simulink model "Pi_si_perturbatii"  (R2022b)
settings: Solver=FixedStepAuto  StartTime=0.0  StopTime=2000  FixedStep=0.01  RelTol=1e-3
values from neighbouring files (symbols this model uses):
  C = 5.6    [CalculeProiect.m]
  h0 = 13.97    [CalculeProiect.m]
  h1 = 17.85    [CalculeProiect.m]
  k = 0.024    [CalculeProiect.m]
  k1 = 0.624    [CalculeProiect.m]
  k11 = k2*k2+4*(k-k3)*k1    (= 0.0616266)    [CalculeProiect.m]
  k12 = 8*(k-k3)    (= 0.1968)    [CalculeProiect.m]
  k13 = 2*(k-k3)    (= 0.0492)    [CalculeProiect.m]
  k2 = -0.015    [CalculeProiect.m]
  k3 = -0.0006    [CalculeProiect.m]
  kp = (delta_h/3)/delta_ua    (= 2.58666666667)    [CalculeProiect.m]
  q0 = 20.97    [CalculeProiect.m]
undefined symbols (not defined in the file or in its folder): ki
libraries: slpidlib x3
settings Model: Creator=denis  LastModifiedBy=denis

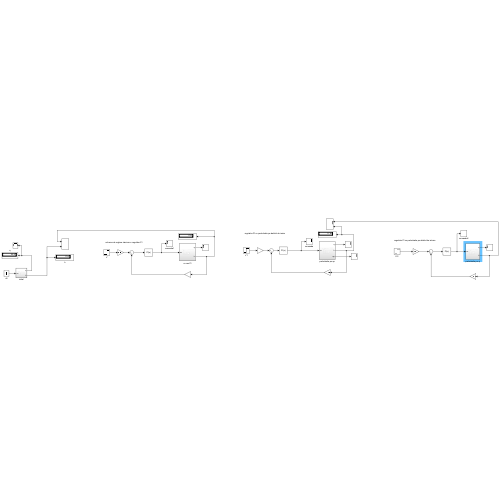
[thumbnail: Simulink's stored preview of the top-level diagram]
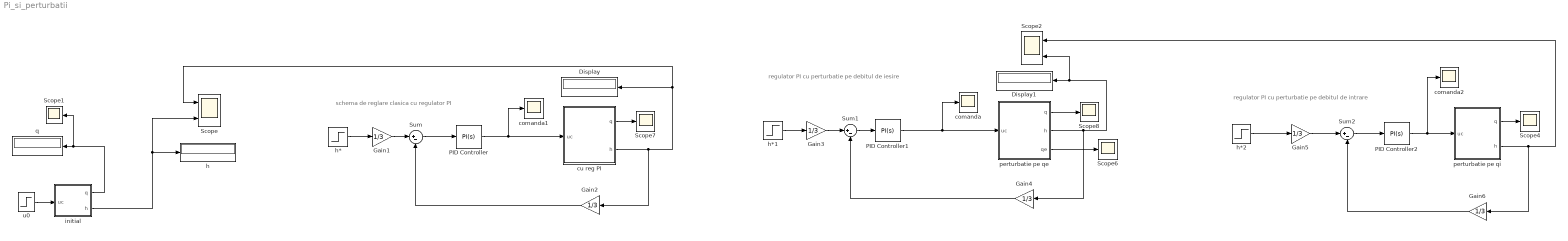
== system Pi_si_perturbatii ==
  note: schema de reglare clasica cu regulator PI
  note: regulator PI cu perturbatie pe debitul de iesire
  note: regulator PI cu perturbatie pe debitul de intrare
  Display : Display
  Display1 : Display
  Gain{1..6} (6 alike) : Gain  Gain=1/3
  PID Controller : slpidlib/PID Controller  Controller=PI  Form=Parallel  TimeDomain=Continuous-time  UseExternalTs=off  SampleTime=-1  IntegratorMethod=Forward Euler  FilterMethod=Forward Euler  ControllerParametersSource=internal  P=kp  I=ki  UseKiTs=off  D=0  N=100  UseFilter=on  TunerSelectOption=Transfer Function Based (PID Tuner App)  InitialConditionSource=internal  InitialConditionForIntegrator=4.4  InitialConditionForFilter=0  DifferentiatorICPrevScaledInput=0  ExternalReset=none  TrackingMode=off  Kt=1  LimitOutput=off  SatLimitsSource=internal  UpperSaturationLimit=inf  LowerSaturationLimit=-inf  LinearizeAsGain=on  AntiWindupMode=none  Kb=1  LimitIntegrator=off  UpperIntegratorSaturationLimit=inf  LowerIntegratorSaturationLimit=-inf  POutMin=[]  POutMax=[]  IOutMin=[]  IOutMax=[]  DOutMin=[]  DOutMax=[]  NOutMin=[]  NOutMax=[]  SumOutMin=[]  SumOutMax=[]  SaturationOutMin=[]  SaturationOutMax=[]  PParamMin=[]  PParamMax=[]  IParamMin=[]  IParamMax=[]  DParamMin=[]  DParamMax=[]  NParamMin=[]  NParamMax=[]  KbParamMin=[]  KbParamMax=[]  KtParamMin=[]  KtParamMax=[]  KbOutMin=[]  KbOutMax=[]  KtOutMin=[]  KtOutMax=[]  IntegratorOutMin=[]  IntegratorOutMax=[]  FilterOutMin=[]  FilterOutMax=[]  SumI1OutMin=[]  SumI1OutMax=[]  SumI2OutMin=[]  SumI2OutMax=[]  SumI3OutMin=[]  SumI3OutMax=[]  SumI4OutMin=[]  SumI4OutMax=[]  SumDOutMin=[]  SumDOutMax=[]  DifferentiatorOutMin=[]  DifferentiatorOutMax=[]  FilterDiffOutCoefMin=[]  FilterDiffOutCoefMax=[]  ReciprocalOutMin=[]  ReciprocalOutMax=[]  SumDenOutMin=[]  SumDenOutMax=[]  SumNumOutMin=[]  SumNumOutMax=[]  DivideOutMin=[]  DivideOutMax=[]  UdiffTsProdOutMin=[]  UdiffTsProdOutMax=[]  NTsProdOutMin=[]  NTsProdOutMax=[]  UintegralTsProdOutMin=[]  UintegralTsProdOutMax=[]  UngainTsProdOutMin=[]  UngainTsProdOutMax=[]  ClampingZeroOutDataTypeStr=Inherit: Inherit via back propagation  ClampingZeroOutMin=[]  ClampingZeroOutMax=[]  FilterDenConstantOutDataTypeStr=Inherit: Inherit via back propagation  FilterDenConstantOutMin=[]  FilterDenConstantOutMax=[]  PCopyOutDataTypeStr=Inherit: Inherit via back propagation  PCopyOutMin=[]  PCopyOutMax=[]  NCopyOutDataTypeStr=Inherit: Inherit via back propagation  NCopyOutMin=[]  NCopyOutMax=[]  IntegratorContinuousStateAttributes=''  IntegratorStateMustResolveToSignalObject=off  IntegratorRTWStateStorageClass=Auto  FilterContinuousStateAttributes=''  FilterStateMustResolveToSignalObject=off  FilterRTWStateStorageClass=Auto  ParallelPVariant=InternalParameters  IdealPVariant=Disabled  IVariant=InternalParameters  DVariant=Disabled  IntegratorVariant=Continuous  SatVariant=Disabled  AWVariant=Passthrough  PCopyVariant=Disabled  TRVariant=Disabled  FdbkBlocksVariant=Forward  IdealPFdbkVariant=Disabled  SatFdbkVariant=Disabled  DerivativeFilterVariant=Disabled  NVariant=Disabled  NCopyVariant=Disabled_SignalSpec  FilterICVariant=Disabled  IntegratorICVariant=InternalICs  ExternalResetVariant=Disabled  TRSumVariant=Passthrough  SumFdbkVariant=Disabled  SumVariant=Sum_PI  TsampFilterVariant=InternalTs  TsampNgainVariant=Passthrough  TsampIntegralVariant=Passthrough  ExternalSaturationOutDataTypeStr=Inherit: Same as second input
  PID Controller1 : slpidlib/PID Controller  Controller=PI  Form=Parallel  TimeDomain=Continuous-time  UseExternalTs=off  SampleTime=-1  IntegratorMethod=Forward Euler  FilterMethod=Forward Euler  ControllerParametersSource=internal  P=kp  I=ki  UseKiTs=off  D=0  N=100  UseFilter=on  TunerSelectOption=Transfer Function Based (PID Tuner App)  InitialConditionSource=internal  InitialConditionForIntegrator=4.4  InitialConditionForFilter=0  DifferentiatorICPrevScaledInput=0  ExternalReset=none  TrackingMode=off  Kt=1  LimitOutput=off  SatLimitsSource=internal  UpperSaturationLimit=inf  LowerSaturationLimit=-inf  LinearizeAsGain=on  AntiWindupMode=none  Kb=1  LimitIntegrator=off  UpperIntegratorSaturationLimit=inf  LowerIntegratorSaturationLimit=-inf  POutMin=[]  POutMax=[]  IOutMin=[]  IOutMax=[]  DOutMin=[]  DOutMax=[]  NOutMin=[]  NOutMax=[]  SumOutMin=[]  SumOutMax=[]  SaturationOutMin=[]  SaturationOutMax=[]  PParamMin=[]  PParamMax=[]  IParamMin=[]  IParamMax=[]  DParamMin=[]  DParamMax=[]  NParamMin=[]  NParamMax=[]  KbParamMin=[]  KbParamMax=[]  KtParamMin=[]  KtParamMax=[]  KbOutMin=[]  KbOutMax=[]  KtOutMin=[]  KtOutMax=[]  IntegratorOutMin=[]  IntegratorOutMax=[]  FilterOutMin=[]  FilterOutMax=[]  SumI1OutMin=[]  SumI1OutMax=[]  SumI2OutMin=[]  SumI2OutMax=[]  SumI3OutMin=[]  SumI3OutMax=[]  SumI4OutMin=[]  SumI4OutMax=[]  SumDOutMin=[]  SumDOutMax=[]  DifferentiatorOutMin=[]  DifferentiatorOutMax=[]  FilterDiffOutCoefMin=[]  FilterDiffOutCoefMax=[]  ReciprocalOutMin=[]  ReciprocalOutMax=[]  SumDenOutMin=[]  SumDenOutMax=[]  SumNumOutMin=[]  SumNumOutMax=[]  DivideOutMin=[]  DivideOutMax=[]  UdiffTsProdOutMin=[]  UdiffTsProdOutMax=[]  NTsProdOutMin=[]  NTsProdOutMax=[]  UintegralTsProdOutMin=[]  UintegralTsProdOutMax=[]  UngainTsProdOutMin=[]  UngainTsProdOutMax=[]  ClampingZeroOutDataTypeStr=Inherit: Inherit via back propagation  ClampingZeroOutMin=[]  ClampingZeroOutMax=[]  FilterDenConstantOutDataTypeStr=Inherit: Inherit via back propagation  FilterDenConstantOutMin=[]  FilterDenConstantOutMax=[]  PCopyOutDataTypeStr=Inherit: Inherit via back propagation  PCopyOutMin=[]  PCopyOutMax=[]  NCopyOutDataTypeStr=Inherit: Inherit via back propagation  NCopyOutMin=[]  NCopyOutMax=[]  IntegratorContinuousStateAttributes=''  IntegratorStateMustResolveToSignalObject=off  IntegratorRTWStateStorageClass=Auto  FilterContinuousStateAttributes=''  FilterStateMustResolveToSignalObject=off  FilterRTWStateStorageClass=Auto  ParallelPVariant=InternalParameters  IdealPVariant=Disabled  IVariant=InternalParameters  DVariant=Disabled  IntegratorVariant=Continuous  SatVariant=Disabled  AWVariant=Passthrough  PCopyVariant=Disabled  TRVariant=Disabled  FdbkBlocksVariant=Forward  IdealPFdbkVariant=Disabled  SatFdbkVariant=Disabled  DerivativeFilterVariant=Disabled  NVariant=Disabled  NCopyVariant=Disabled_SignalSpec  FilterICVariant=Disabled  IntegratorICVariant=InternalICs  ExternalResetVariant=Disabled  TRSumVariant=Passthrough  SumFdbkVariant=Disabled  SumVariant=Sum_PI  TsampFilterVariant=InternalTs  TsampNgainVariant=Passthrough  TsampIntegralVariant=Passthrough  ExternalSaturationOutDataTypeStr=Inherit: Same as second input
  PID Controller2 : slpidlib/PID Controller  Controller=PI  Form=Parallel  TimeDomain=Continuous-time  UseExternalTs=off  SampleTime=-1  IntegratorMethod=Forward Euler  FilterMethod=Forward Euler  ControllerParametersSource=internal  P=kp  I=ki  UseKiTs=off  D=0  N=100  UseFilter=on  TunerSelectOption=Transfer Function Based (PID Tuner App)  InitialConditionSource=internal  InitialConditionForIntegrator=4.4  InitialConditionForFilter=0  DifferentiatorICPrevScaledInput=0  ExternalReset=none  TrackingMode=off  Kt=1  LimitOutput=off  SatLimitsSource=internal  UpperSaturationLimit=inf  LowerSaturationLimit=-inf  LinearizeAsGain=on  AntiWindupMode=none  Kb=1  LimitIntegrator=off  UpperIntegratorSaturationLimit=inf  LowerIntegratorSaturationLimit=-inf  POutMin=[]  POutMax=[]  IOutMin=[]  IOutMax=[]  DOutMin=[]  DOutMax=[]  NOutMin=[]  NOutMax=[]  SumOutMin=[]  SumOutMax=[]  SaturationOutMin=[]  SaturationOutMax=[]  PParamMin=[]  PParamMax=[]  IParamMin=[]  IParamMax=[]  DParamMin=[]  DParamMax=[]  NParamMin=[]  NParamMax=[]  KbParamMin=[]  KbParamMax=[]  KtParamMin=[]  KtParamMax=[]  KbOutMin=[]  KbOutMax=[]  KtOutMin=[]  KtOutMax=[]  IntegratorOutMin=[]  IntegratorOutMax=[]  FilterOutMin=[]  FilterOutMax=[]  SumI1OutMin=[]  SumI1OutMax=[]  SumI2OutMin=[]  SumI2OutMax=[]  SumI3OutMin=[]  SumI3OutMax=[]  SumI4OutMin=[]  SumI4OutMax=[]  SumDOutMin=[]  SumDOutMax=[]  DifferentiatorOutMin=[]  DifferentiatorOutMax=[]  FilterDiffOutCoefMin=[]  FilterDiffOutCoefMax=[]  ReciprocalOutMin=[]  ReciprocalOutMax=[]  SumDenOutMin=[]  SumDenOutMax=[]  SumNumOutMin=[]  SumNumOutMax=[]  DivideOutMin=[]  DivideOutMax=[]  UdiffTsProdOutMin=[]  UdiffTsProdOutMax=[]  NTsProdOutMin=[]  NTsProdOutMax=[]  UintegralTsProdOutMin=[]  UintegralTsProdOutMax=[]  UngainTsProdOutMin=[]  UngainTsProdOutMax=[]  ClampingZeroOutDataTypeStr=Inherit: Inherit via back propagation  ClampingZeroOutMin=[]  ClampingZeroOutMax=[]  FilterDenConstantOutDataTypeStr=Inherit: Inherit via back propagation  FilterDenConstantOutMin=[]  FilterDenConstantOutMax=[]  PCopyOutDataTypeStr=Inherit: Inherit via back propagation  PCopyOutMin=[]  PCopyOutMax=[]  NCopyOutDataTypeStr=Inherit: Inherit via back propagation  NCopyOutMin=[]  NCopyOutMax=[]  IntegratorContinuousStateAttributes=''  IntegratorStateMustResolveToSignalObject=off  IntegratorRTWStateStorageClass=Auto  FilterContinuousStateAttributes=''  FilterStateMustResolveToSignalObject=off  FilterRTWStateStorageClass=Auto  ParallelPVariant=InternalParameters  IdealPVariant=Disabled  IVariant=InternalParameters  DVariant=Disabled  IntegratorVariant=Continuous  SatVariant=Disabled  AWVariant=Passthrough  PCopyVariant=Disabled  TRVariant=Disabled  FdbkBlocksVariant=Forward  IdealPFdbkVariant=Disabled  SatFdbkVariant=Disabled  DerivativeFilterVariant=Disabled  NVariant=Disabled  NCopyVariant=Disabled_SignalSpec  FilterICVariant=Disabled  IntegratorICVariant=InternalICs  ExternalResetVariant=Disabled  TRSumVariant=Passthrough  SumFdbkVariant=Disabled  SumVariant=Sum_PI  TsampFilterVariant=InternalTs  TsampNgainVariant=Passthrough  TsampIntegralVariant=Passthrough  ExternalSaturationOutDataTypeStr=Inherit: Same as second input
  Scope : Scope  NumInputPorts=2
  Scope{1,4,6..8} (5 alike) : Scope
  Scope2 : Scope  NumInputPorts=2
  Sum : Sum  Inputs=|+-
  Sum1 : Sum  Inputs=|+-
  Sum2 : Sum  Inputs=|+-
  comanda : Scope
  comanda1 : Scope
  comanda2 : Scope
  cu reg PI : Subsystem
  h : Display
  h* : Step  Time=0  Before=h0  After=h1  SampleTime=0
  h*1 : Step  Time=0  Before=h0  After=h1  SampleTime=0
  h*2 : Step  Time=0  Before=h0  After=h1  SampleTime=0
  initial : Subsystem
  perturbatie pe qe : Subsystem
  perturbatie pe qi : Subsystem
  q : Display
  u0 : Step  Time=0  Before=4.4  After=4.9  SampleTime=0
  wires:
  Sum2/1 -> PID Controller2/1
  h*2/1 -> Gain5/1
  perturbatie pe qe/1(q) -> Scope8/1
  perturbatie pe qi/1(q) -> Scope4/1
  Gain5/1 -> Sum2/1
  Gain3/1 -> Sum1/1
  initial/2(h) -> Scope/2, h/1
  Sum/1 -> PID Controller/1
  Sum1/1 -> PID Controller1/1
  PID Controller/1 -> comanda1/1, cu reg PI/1(uc)
  h*1/1 -> Gain3/1
  Gain6/1 -> Sum2/2
  perturbatie pe qe/2(h) -> Gain4/1, Scope2/2, Display1/1
  PID Controller1/1 -> comanda/1, perturbatie pe qe/1(uc)
  Gain4/1 -> Sum1/2
  perturbatie pe qe/3(qe) -> Scope6/1
  h*/1 -> Gain1/1
  Gain2/1 -> Sum/2
  perturbatie pe qi/2(h) -> Scope2/1, Gain6/1
  u0/1 -> initial/1(uc)
  cu reg PI/2(h) -> Gain2/1, Display/1, Scope/1
  cu reg PI/1(q) -> Scope7/1
  Gain1/1 -> Sum/1
  PID Controller2/1 -> comanda2/1, perturbatie pe qi/1(uc)
  initial/1(q) -> Scope1/1, q/1

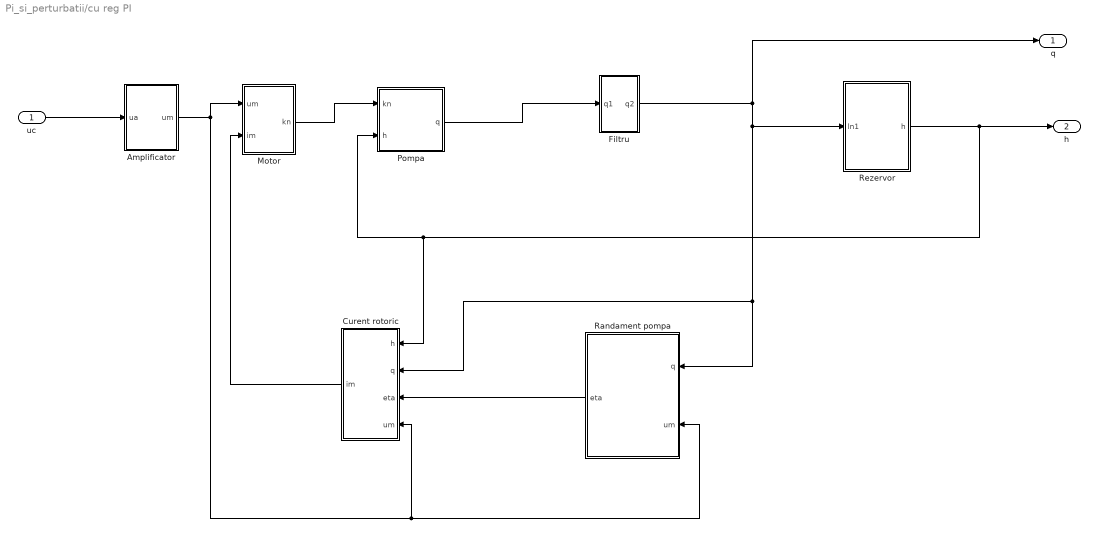
== system Pi_si_perturbatii/cu reg PI ==
  uc : Inport
  Amplificator : Subsystem
  Curent rotoric : Subsystem
  Filtru : Subsystem
  Motor : Subsystem
  Pompa : Subsystem
  Randament pompa : Subsystem
  Rezervor : Subsystem
  q : Outport
  h : Outport  Port=2
  wires:
  Filtru/1(q2) -> Curent rotoric/2(q), Randament pompa/1(q), Rezervor/1(ln1), q/1
  Rezervor/1(h) -> h/1, Curent rotoric/1(h), Pompa/2(h)
  Motor/1(kn) -> Pompa/1(kn)
  Curent rotoric/1(im) -> Motor/2(im)
  Amplificator/1(um) -> Motor/1(um), Curent rotoric/4(um), Randament pompa/2(um)
  uc/1 -> Amplificator/1(ua)
  Randament pompa/1(eta) -> Curent rotoric/3(eta)
  Pompa/1(q) -> Filtru/1(q1)

== system Pi_si_perturbatii/initial ==
  uc : Inport
  Amplificator : Subsystem
  Curent rotoric : Subsystem
  Filtru : Subsystem
  Motor : Subsystem
  Pompa : Subsystem
  Randament pompa : Subsystem
  Rezervor : Subsystem
  q : Outport
  h : Outport  Port=2
  wires:
  Filtru/1(q2) -> Curent rotoric/2(q), Randament pompa/1(q), Rezervor/1(ln1), q/1
  Rezervor/1(h) -> h/1, Curent rotoric/1(h), Pompa/2(h)
  Motor/1(kn) -> Pompa/1(kn)
  Curent rotoric/1(im) -> Motor/2(im)
  Amplificator/1(um) -> Motor/1(um), Curent rotoric/4(um), Randament pompa/2(um)
  uc/1 -> Amplificator/1(ua)
  Randament pompa/1(eta) -> Curent rotoric/3(eta)
  Pompa/1(q) -> Filtru/1(q1)

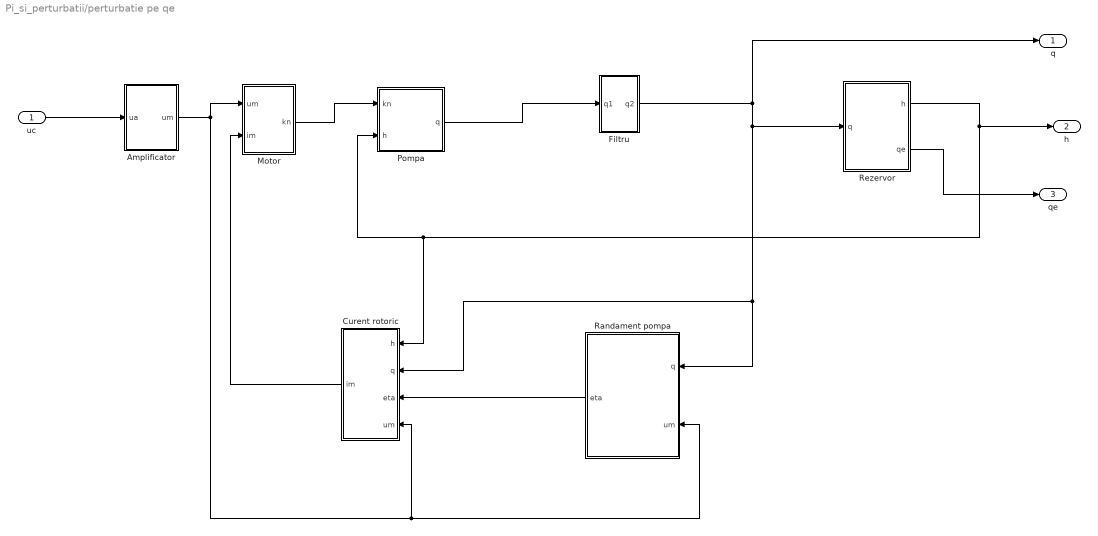
== system Pi_si_perturbatii/perturbatie pe qe ==
  uc : Inport
  Amplificator : Subsystem
  Curent rotoric : Subsystem
  Filtru : Subsystem
  Motor : Subsystem
  Pompa : Subsystem
  Randament pompa : Subsystem
  Rezervor : Subsystem
  q : Outport
  h : Outport  Port=2
  qe : Outport  Port=3
  wires:
  Filtru/1(q2) -> Curent rotoric/2(q), Randament pompa/1(q), Rezervor/1(q), q/1
  Rezervor/1(h) -> h/1, Curent rotoric/1(h), Pompa/2(h)
  Motor/1(kn) -> Pompa/1(kn)
  Curent rotoric/1(im) -> Motor/2(im)
  Amplificator/1(um) -> Motor/1(um), Curent rotoric/4(um), Randament pompa/2(um)
  uc/1 -> Amplificator/1(ua)
  Randament pompa/1(eta) -> Curent rotoric/3(eta)
  Pompa/1(q) -> Filtru/1(q1)
  Rezervor/2(qe) -> qe/1

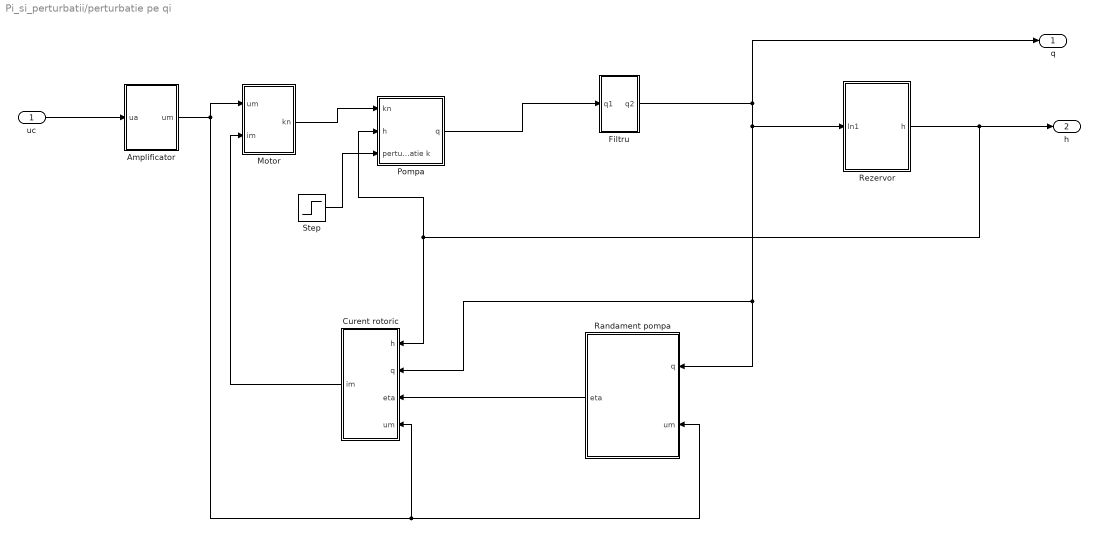
== system Pi_si_perturbatii/perturbatie pe qi ==
  uc : Inport
  Amplificator : Subsystem
  Curent rotoric : Subsystem
  Filtru : Subsystem
  Motor : Subsystem
  Pompa : Subsystem
  Randament pompa : Subsystem
  Rezervor : Subsystem
  Step : Step  Time=250  After=0.03  SampleTime=0
  q : Outport
  h : Outport  Port=2
  wires:
  Filtru/1(q2) -> Curent rotoric/2(q), Randament pompa/1(q), Rezervor/1(ln1), q/1
  Rezervor/1(h) -> h/1, Pompa/2(h), Curent rotoric/1(h)
  Motor/1(kn) -> Pompa/1(kn)
  Curent rotoric/1(im) -> Motor/2(im)
  Amplificator/1(um) -> Motor/1(um), Curent rotoric/4(um), Randament pompa/2(um)
  uc/1 -> Amplificator/1(ua)
  Randament pompa/1(eta) -> Curent rotoric/3(eta)
  Pompa/1(q) -> Filtru/1(q1)
  Step/1 -> Pompa/3(perturbatie k)

== system Pi_si_perturbatii/cu reg PI/Amplificator ==
  ua : Inport
  Constant : Constant  Value=8.1
  Gain : Gain  Gain=2.2
  Gain1 : Gain  Gain=5
  Gain2 : Gain  Gain=2.2
  Saturation : Saturate  UpperLimit=22  LowerLimit=0
  Sum : Sum  Inputs=|++
  Sum1 : Sum  Inputs=|+-
  Switch : Switch  Criteria=u2 > Threshold  Threshold=8.1  SaturateOnIntegerOverflow=off  InputSameDT=off
  um : Outport
  wires:
  Gain/1 -> Switch/3
  Sum1/1 -> Gain1/1
  ua/1 -> Gain/1, Sum1/1, Gain2/1, Switch/2
  Switch/1 -> Saturation/1
  Gain1/1 -> Sum/2
  Saturation/1 -> um/1
  Constant/1 -> Sum1/2
  Gain2/1 -> Sum/1
  Sum/1 -> Switch/1

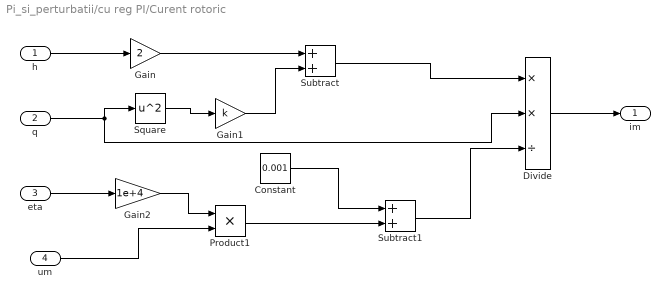
== system Pi_si_perturbatii/cu reg PI/Curent rotoric ==
  h : Inport
  q : Inport  Port=2
  eta : Inport  Port=3
  um : Inport  Port=4
  Constant : Constant  Value=0.001
  Divide : Product  Inputs=**/
  Gain : Gain  Gain=2
  Gain1 : Gain  Gain=k
  Gain2 : Gain  Gain=1e+4
  Product1 : Product
  Square : Math  Operator=square
  Subtract : Sum
  Subtract1 : Sum
  im : Outport
  wires:
  h/1 -> Gain/1
  Divide/1 -> im/1
  q/1 -> Divide/2, Square/1
  eta/1 -> Gain2/1
  um/1 -> Product1/2
  Gain2/1 -> Product1/1
  Subtract/1 -> Divide/1
  Constant/1 -> Subtract1/1
  Product1/1 -> Subtract1/2
  Subtract1/1 -> Divide/3
  Gain/1 -> Subtract/1
  Gain1/1 -> Subtract/2
  Square/1 -> Gain1/1

== system Pi_si_perturbatii/cu reg PI/Filtru ==
  q1 : Inport
  Integrator1 : Integrator  InitialCondition=q0
  Sum1 : Sum  Inputs=|+-
  q2 : Outport
  wires:
  Integrator1/1 -> q2/1, Sum1/2
  q1/1 -> Sum1/1
  Sum1/1 -> Integrator1/1

== system Pi_si_perturbatii/cu reg PI/Motor ==
  um : Inport
  im : Inport  Port=2
  Add : Sum  Inputs=+-
  Rm : Gain  Gain=3
  kn : Outport
  wires:
  Rm/1 -> Add/2
  um/1 -> Add/1
  im/1 -> Rm/1
  Add/1 -> kn/1

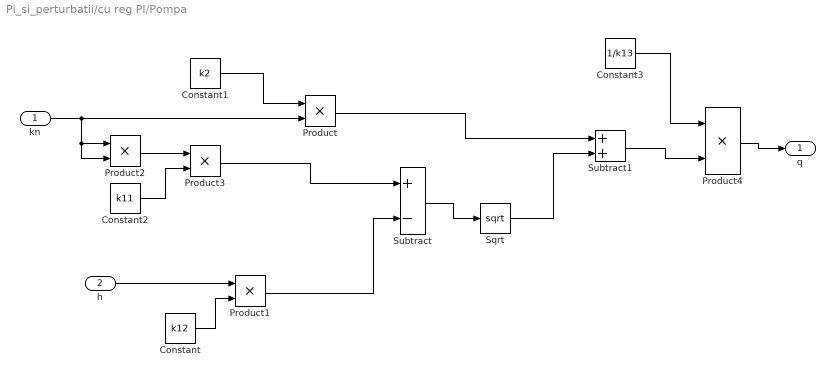
== system Pi_si_perturbatii/cu reg PI/Pompa ==
  kn : Inport
  h : Inport  Port=2
  Constant : Constant  Value=k12
  Constant1 : Constant  Value=k2
  Constant2 : Constant  Value=k11
  Constant3 : Constant  Value=1/k13
  Product{,1..4} (5 alike) : Product
  Sqrt : Sqrt
  Subtract : Sum  Inputs=+-
  Subtract1 : Sum
  q : Outport
  wires:
  Subtract/1 -> Sqrt/1
  Sqrt/1 -> Subtract1/2
  h/1 -> Product1/1
  Product1/1 -> Subtract/2
  Constant/1 -> Product1/2
  Constant1/1 -> Product/1
  kn/1 -> Product2/2, Product2/1, Product/2
  Product/1 -> Subtract1/1
  Product2/1 -> Product3/1
  Constant2/1 -> Product3/2
  Product3/1 -> Subtract/1
  Constant3/1 -> Product4/1
  Subtract1/1 -> Product4/2
  Product4/1 -> q/1

== system Pi_si_perturbatii/cu reg PI/Randament pompa ==
  q : Inport
  um : Inport  Port=2
  Gain : Gain  Gain=8e-5
  Product : Product
  eta : Outport
  wires:
  um/1 -> Gain/1
  Gain/1 -> Product/2
  q/1 -> Product/1
  Product/1 -> eta/1

== system Pi_si_perturbatii/cu reg PI/Rezervor ==
  ln1 : Inport
  Gain : Gain  Gain=1/332.5
  Gain1 : Gain  Gain=C
  Integrator1 : Integrator  InitialCondition=h0
  Sqrt : Sqrt
  Sum1 : Sum  Inputs=|+-
  h : Outport
  wires:
  Gain/1 -> Integrator1/1
  Integrator1/1 -> Sqrt/1, h/1
  Sum1/1 -> Gain/1
  ln1/1 -> Sum1/1
  Sqrt/1 -> Gain1/1
  Gain1/1 -> Sum1/2

== system Pi_si_perturbatii/initial/Amplificator ==
  ua : Inport
  Constant : Constant  Value=8.1
  Gain : Gain  Gain=2.2
  Gain1 : Gain  Gain=5
  Gain2 : Gain  Gain=2.2
  Saturation : Saturate  UpperLimit=22  LowerLimit=0
  Sum : Sum  Inputs=|++
  Sum1 : Sum  Inputs=|+-
  Switch : Switch  Criteria=u2 > Threshold  Threshold=8.1  SaturateOnIntegerOverflow=off  InputSameDT=off
  um : Outport
  wires:
  Gain/1 -> Switch/3
  Sum1/1 -> Gain1/1
  ua/1 -> Gain/1, Sum1/1, Gain2/1, Switch/2
  Switch/1 -> Saturation/1
  Gain1/1 -> Sum/2
  Saturation/1 -> um/1
  Constant/1 -> Sum1/2
  Gain2/1 -> Sum/1
  Sum/1 -> Switch/1

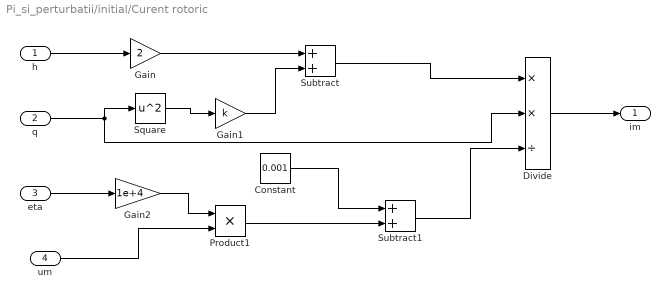
== system Pi_si_perturbatii/initial/Curent rotoric ==
  h : Inport
  q : Inport  Port=2
  eta : Inport  Port=3
  um : Inport  Port=4
  Constant : Constant  Value=0.001
  Divide : Product  Inputs=**/
  Gain : Gain  Gain=2
  Gain1 : Gain  Gain=k
  Gain2 : Gain  Gain=1e+4
  Product1 : Product
  Square : Math  Operator=square
  Subtract : Sum
  Subtract1 : Sum
  im : Outport
  wires:
  h/1 -> Gain/1
  Divide/1 -> im/1
  q/1 -> Divide/2, Square/1
  eta/1 -> Gain2/1
  um/1 -> Product1/2
  Gain2/1 -> Product1/1
  Subtract/1 -> Divide/1
  Constant/1 -> Subtract1/1
  Product1/1 -> Subtract1/2
  Subtract1/1 -> Divide/3
  Gain/1 -> Subtract/1
  Gain1/1 -> Subtract/2
  Square/1 -> Gain1/1

== system Pi_si_perturbatii/initial/Filtru ==
  q1 : Inport
  Integrator1 : Integrator  InitialCondition=q0
  Sum1 : Sum  Inputs=|+-
  q2 : Outport
  wires:
  Integrator1/1 -> q2/1, Sum1/2
  q1/1 -> Sum1/1
  Sum1/1 -> Integrator1/1

== system Pi_si_perturbatii/initial/Motor ==
  um : Inport
  im : Inport  Port=2
  Add : Sum  Inputs=+-
  Rm : Gain  Gain=3
  kn : Outport
  wires:
  Rm/1 -> Add/2
  um/1 -> Add/1
  im/1 -> Rm/1
  Add/1 -> kn/1

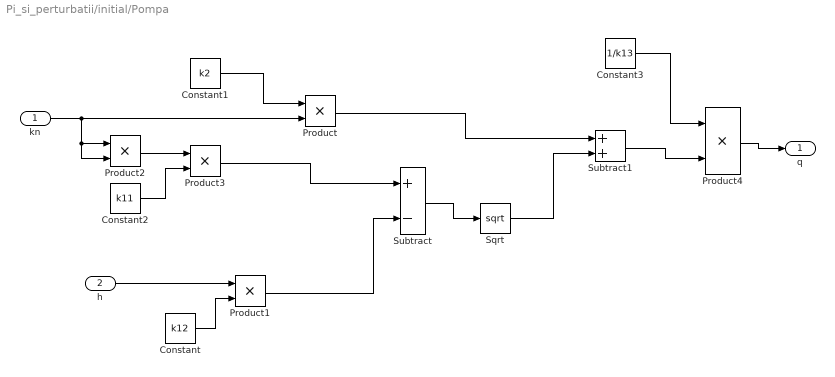
== system Pi_si_perturbatii/initial/Pompa ==
  kn : Inport
  h : Inport  Port=2
  Constant : Constant  Value=k12
  Constant1 : Constant  Value=k2
  Constant2 : Constant  Value=k11
  Constant3 : Constant  Value=1/k13
  Product{,1..4} (5 alike) : Product
  Sqrt : Sqrt
  Subtract : Sum  Inputs=+-
  Subtract1 : Sum
  q : Outport
  wires:
  Subtract/1 -> Sqrt/1
  Sqrt/1 -> Subtract1/2
  h/1 -> Product1/1
  Product1/1 -> Subtract/2
  Constant/1 -> Product1/2
  Constant1/1 -> Product/1
  kn/1 -> Product2/2, Product2/1, Product/2
  Product/1 -> Subtract1/1
  Product2/1 -> Product3/1
  Constant2/1 -> Product3/2
  Product3/1 -> Subtract/1
  Constant3/1 -> Product4/1
  Subtract1/1 -> Product4/2
  Product4/1 -> q/1

== system Pi_si_perturbatii/initial/Randament pompa ==
  q : Inport
  um : Inport  Port=2
  Gain : Gain  Gain=8e-5
  Product : Product
  eta : Outport
  wires:
  um/1 -> Gain/1
  Gain/1 -> Product/2
  q/1 -> Product/1
  Product/1 -> eta/1

== system Pi_si_perturbatii/initial/Rezervor ==
  ln1 : Inport
  Gain : Gain  Gain=1/332.5
  Gain1 : Gain  Gain=C
  Integrator1 : Integrator  InitialCondition=h0
  Sqrt : Sqrt
  Sum1 : Sum  Inputs=|+-
  h : Outport
  wires:
  Gain/1 -> Integrator1/1
  Integrator1/1 -> Sqrt/1, h/1
  Sum1/1 -> Gain/1
  ln1/1 -> Sum1/1
  Sqrt/1 -> Gain1/1
  Gain1/1 -> Sum1/2

== system Pi_si_perturbatii/perturbatie pe qe/Amplificator ==
  ua : Inport
  Constant : Constant  Value=8.1
  Gain : Gain  Gain=2.2
  Gain1 : Gain  Gain=5
  Gain2 : Gain  Gain=2.2
  Saturation : Saturate  UpperLimit=22  LowerLimit=0
  Sum : Sum  Inputs=|++
  Sum1 : Sum  Inputs=|+-
  Switch : Switch  Criteria=u2 > Threshold  Threshold=8.1  SaturateOnIntegerOverflow=off  InputSameDT=off
  um : Outport
  wires:
  Gain/1 -> Switch/3
  Sum1/1 -> Gain1/1
  ua/1 -> Gain/1, Sum1/1, Gain2/1, Switch/2
  Switch/1 -> Saturation/1
  Gain1/1 -> Sum/2
  Saturation/1 -> um/1
  Constant/1 -> Sum1/2
  Gain2/1 -> Sum/1
  Sum/1 -> Switch/1

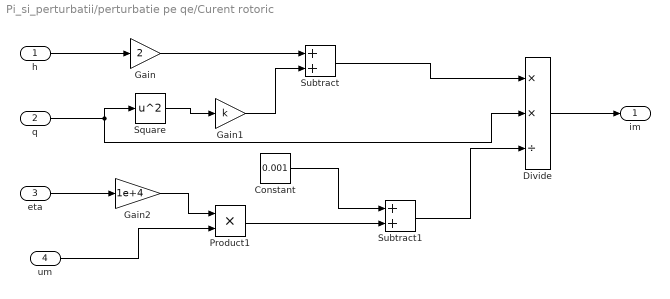
== system Pi_si_perturbatii/perturbatie pe qe/Curent rotoric ==
  h : Inport
  q : Inport  Port=2
  eta : Inport  Port=3
  um : Inport  Port=4
  Constant : Constant  Value=0.001
  Divide : Product  Inputs=**/
  Gain : Gain  Gain=2
  Gain1 : Gain  Gain=k
  Gain2 : Gain  Gain=1e+4
  Product1 : Product
  Square : Math  Operator=square
  Subtract : Sum
  Subtract1 : Sum
  im : Outport
  wires:
  h/1 -> Gain/1
  Divide/1 -> im/1
  q/1 -> Divide/2, Square/1
  eta/1 -> Gain2/1
  um/1 -> Product1/2
  Gain2/1 -> Product1/1
  Subtract/1 -> Divide/1
  Constant/1 -> Subtract1/1
  Product1/1 -> Subtract1/2
  Subtract1/1 -> Divide/3
  Gain/1 -> Subtract/1
  Gain1/1 -> Subtract/2
  Square/1 -> Gain1/1

== system Pi_si_perturbatii/perturbatie pe qe/Filtru ==
  q1 : Inport
  Integrator1 : Integrator  InitialCondition=q0
  Sum1 : Sum  Inputs=|+-
  q2 : Outport
  wires:
  Integrator1/1 -> q2/1, Sum1/2
  q1/1 -> Sum1/1
  Sum1/1 -> Integrator1/1

== system Pi_si_perturbatii/perturbatie pe qe/Motor ==
  um : Inport
  im : Inport  Port=2
  Add : Sum  Inputs=+-
  Rm : Gain  Gain=3
  kn : Outport
  wires:
  Rm/1 -> Add/2
  um/1 -> Add/1
  im/1 -> Rm/1
  Add/1 -> kn/1

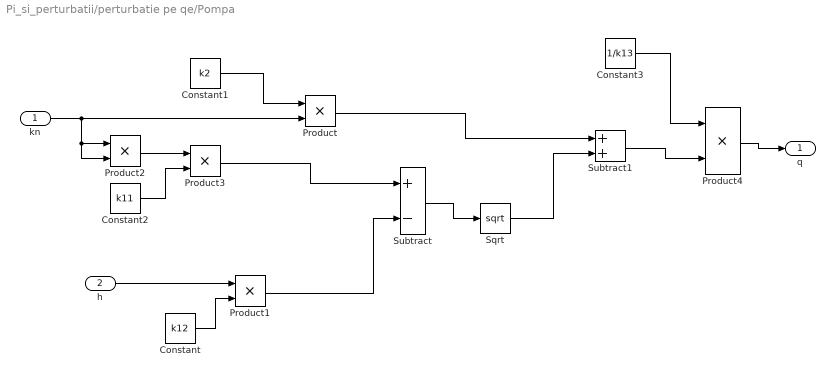
== system Pi_si_perturbatii/perturbatie pe qe/Pompa ==
  kn : Inport
  h : Inport  Port=2
  Constant : Constant  Value=k12
  Constant1 : Constant  Value=k2
  Constant2 : Constant  Value=k11
  Constant3 : Constant  Value=1/k13
  Product{,1..4} (5 alike) : Product
  Sqrt : Sqrt
  Subtract : Sum  Inputs=+-
  Subtract1 : Sum
  q : Outport
  wires:
  Subtract/1 -> Sqrt/1
  Sqrt/1 -> Subtract1/2
  h/1 -> Product1/1
  Product1/1 -> Subtract/2
  Constant/1 -> Product1/2
  Constant1/1 -> Product/1
  kn/1 -> Product2/2, Product2/1, Product/2
  Product/1 -> Subtract1/1
  Product2/1 -> Product3/1
  Constant2/1 -> Product3/2
  Product3/1 -> Subtract/1
  Constant3/1 -> Product4/1
  Subtract1/1 -> Product4/2
  Product4/1 -> q/1

== system Pi_si_perturbatii/perturbatie pe qe/Randament pompa ==
  q : Inport
  um : Inport  Port=2
  Gain : Gain  Gain=8e-5
  Product : Product
  eta : Outport
  wires:
  um/1 -> Gain/1
  Gain/1 -> Product/2
  q/1 -> Product/1
  Product/1 -> eta/1

== system Pi_si_perturbatii/perturbatie pe qe/Rezervor ==
  q : Inport
  C : Step  Time=250  Before=5.6  After=9  SampleTime=0
  Gain : Gain  Gain=1/332.5
  Integrator1 : Integrator  InitialCondition=h0
  Product : Product
  Sqrt : Sqrt
  Sum1 : Sum  Inputs=|+-
  h : Outport
  qe : Outport  Port=2
  wires:
  Gain/1 -> Integrator1/1
  Integrator1/1 -> Sqrt/1, h/1
  Sum1/1 -> Gain/1
  q/1 -> Sum1/1
  Product/1 -> qe/1, Sum1/2
  Sqrt/1 -> Product/1
  C/1 -> Product/2

== system Pi_si_perturbatii/perturbatie pe qi/Amplificator ==
  ua : Inport
  Constant : Constant  Value=8.1
  Gain : Gain  Gain=2.2
  Gain1 : Gain  Gain=5
  Gain2 : Gain  Gain=2.2
  Saturation : Saturate  UpperLimit=22  LowerLimit=0
  Sum : Sum  Inputs=|++
  Sum1 : Sum  Inputs=|+-
  Switch : Switch  Criteria=u2 > Threshold  Threshold=8.1  SaturateOnIntegerOverflow=off  InputSameDT=off
  um : Outport
  wires:
  Gain/1 -> Switch/3
  Sum1/1 -> Gain1/1
  ua/1 -> Gain/1, Sum1/1, Gain2/1, Switch/2
  Switch/1 -> Saturation/1
  Gain1/1 -> Sum/2
  Saturation/1 -> um/1
  Constant/1 -> Sum1/2
  Gain2/1 -> Sum/1
  Sum/1 -> Switch/1

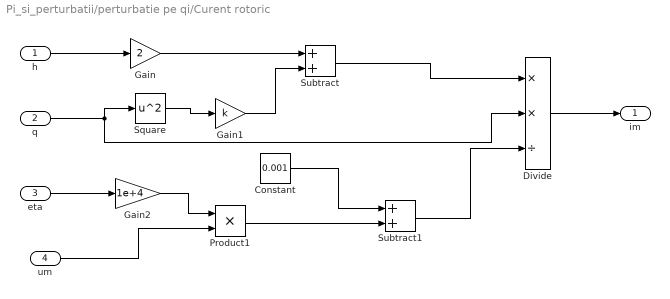
== system Pi_si_perturbatii/perturbatie pe qi/Curent rotoric ==
  h : Inport
  q : Inport  Port=2
  eta : Inport  Port=3
  um : Inport  Port=4
  Constant : Constant  Value=0.001
  Divide : Product  Inputs=**/
  Gain : Gain  Gain=2
  Gain1 : Gain  Gain=k
  Gain2 : Gain  Gain=1e+4
  Product1 : Product
  Square : Math  Operator=square
  Subtract : Sum
  Subtract1 : Sum
  im : Outport
  wires:
  h/1 -> Gain/1
  Divide/1 -> im/1
  q/1 -> Divide/2, Square/1
  eta/1 -> Gain2/1
  um/1 -> Product1/2
  Gain2/1 -> Product1/1
  Subtract/1 -> Divide/1
  Constant/1 -> Subtract1/1
  Product1/1 -> Subtract1/2
  Subtract1/1 -> Divide/3
  Gain/1 -> Subtract/1
  Gain1/1 -> Subtract/2
  Square/1 -> Gain1/1

== system Pi_si_perturbatii/perturbatie pe qi/Filtru ==
  q1 : Inport
  Integrator1 : Integrator  InitialCondition=q0
  Sum1 : Sum  Inputs=|+-
  q2 : Outport
  wires:
  Integrator1/1 -> q2/1, Sum1/2
  q1/1 -> Sum1/1
  Sum1/1 -> Integrator1/1

== system Pi_si_perturbatii/perturbatie pe qi/Motor ==
  um : Inport
  im : Inport  Port=2
  Add : Sum  Inputs=+-
  Rm : Gain  Gain=3
  kn : Outport
  wires:
  Rm/1 -> Add/2
  um/1 -> Add/1
  im/1 -> Rm/1
  Add/1 -> kn/1

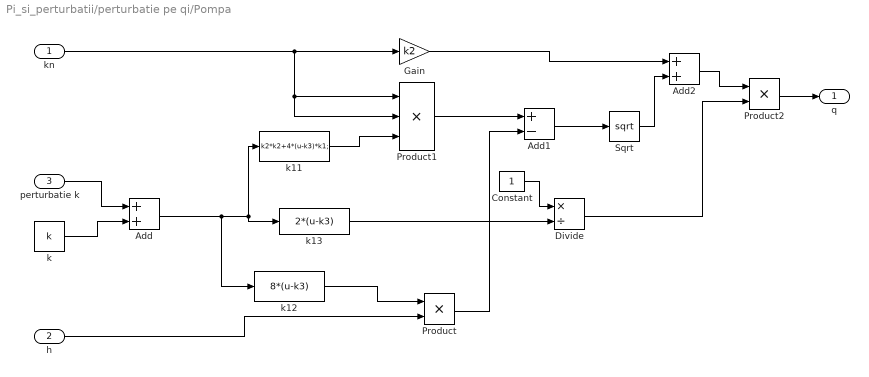
== system Pi_si_perturbatii/perturbatie pe qi/Pompa ==
  kn : Inport
  h : Inport  Port=2
  perturbatie k : Inport  Port=3
  Add : Sum
  Add1 : Sum  Inputs=+-
  Add2 : Sum
  Constant : Constant
  Divide : Product  Inputs=*/
  Gain : Gain  Gain=k2
  Product : Product
  Product1 : Product  Inputs=3
  Product2 : Product
  Sqrt : Sqrt
  k : Constant  Value=k
  k11 : MATLABFcn  MATLABFcn=k2*k2+4*(u-k3)*k1;
  k12 : MATLABFcn  MATLABFcn=8*(u-k3)
  k13 : MATLABFcn  MATLABFcn=2*(u-k3)
  q : Outport
  wires:
  perturbatie k/1 -> Add/1
  k/1 -> Add/2
  k12/1 -> Product/1
  h/1 -> Product/2
  Add/1 -> k12/1, k13/1, k11/1
  k11/1 -> Product1/3
  kn/1 -> Product1/1, Product1/2, Gain/1
  Product1/1 -> Add1/1
  Product/1 -> Add1/2
  Add1/1 -> Sqrt/1
  Gain/1 -> Add2/1
  Sqrt/1 -> Add2/2
  k13/1 -> Divide/2
  Constant/1 -> Divide/1
  Add2/1 -> Product2/1
  Divide/1 -> Product2/2
  Product2/1 -> q/1

== system Pi_si_perturbatii/perturbatie pe qi/Randament pompa ==
  q : Inport
  um : Inport  Port=2
  Gain : Gain  Gain=8e-5
  Product : Product
  eta : Outport
  wires:
  um/1 -> Gain/1
  Gain/1 -> Product/2
  q/1 -> Product/1
  Product/1 -> eta/1

== system Pi_si_perturbatii/perturbatie pe qi/Rezervor ==
  ln1 : Inport
  Gain : Gain  Gain=1/332.5
  Gain1 : Gain  Gain=C
  Integrator1 : Integrator  InitialCondition=h0
  Sqrt : Sqrt
  Sum1 : Sum  Inputs=|+-
  h : Outport
  wires:
  Gain/1 -> Integrator1/1
  Integrator1/1 -> Sqrt/1, h/1
  Sum1/1 -> Gain/1
  ln1/1 -> Sum1/1
  Sqrt/1 -> Gain1/1
  Gain1/1 -> Sum1/2
